simulink model "sampleModel1946"  (R2023a)
settings: Solver=VariableStepAuto  StartTime=0.0  StopTime=10.0  RelTol=1e-3
libraries: hdlsllib x1
settings Model: Creator=user1  LastModifiedBy=user1

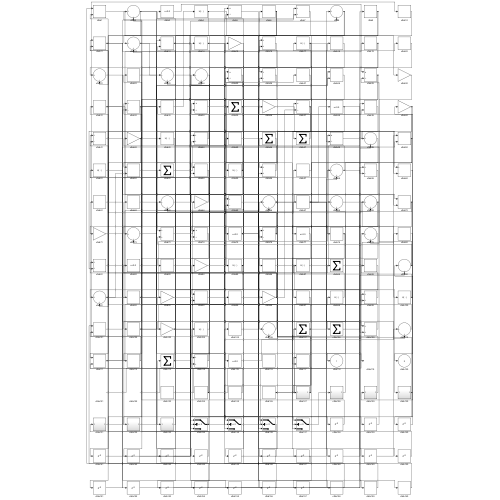
[thumbnail: Simulink's stored preview of the top-level diagram]
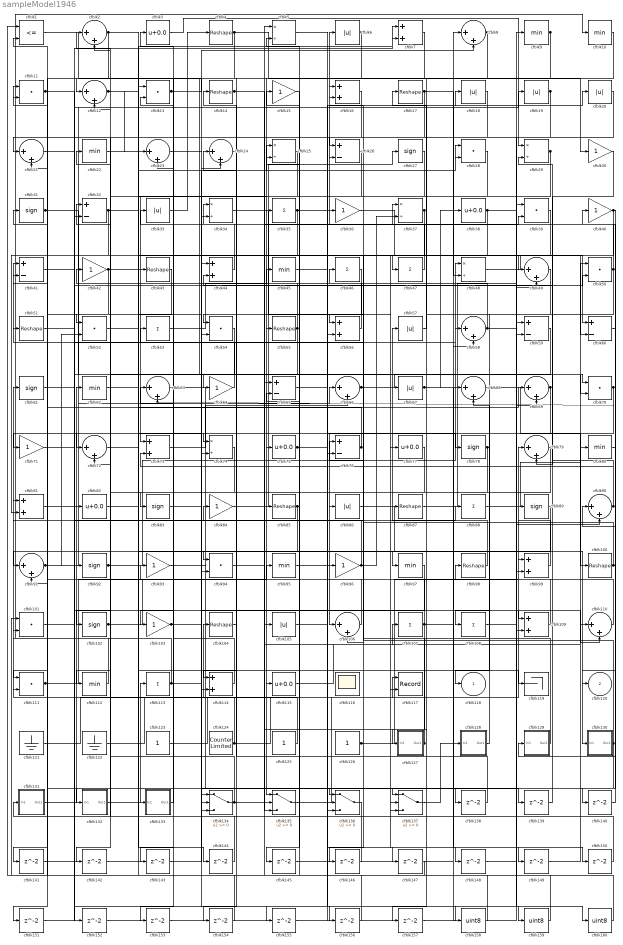
== system sampleModel1946 ==
  cfblk1 : RelationalOperator  Operator=<=  OutDataTypeStr=boolean  InputSameDT=off
  cfblk{9..10,22,45,62,80,95,97,112} (9 alike) : MinMax
  cfblk{4,14,17,43,51,55,85,87,98,100,104} (11 alike) : Reshape
  cfblk{11,13,28,39,50,52,54,70,94,101,111} (11 alike) : DotProduct  OutDataTypeStr=Inherit: Inherit via internal rule
  cfblk{27,31,61,78,83,89,92,102} (8 alike) : Signum
  cfblk{15,30,36,40,42,64,71,84,93,96,103} (11 alike) : Gain
  cfblk{6,18..20,33,57,67,86,105} (9 alike) : Abs  SaturateOnIntegerOverflow=off
  cfblk{2,8,12,21,23..24,49,58,63,66,68..69,72,79,90..91,106,110} (18 alike) : Sum  Inputs=|++
  cfblk{35,46..47,53,88,107..108,113} (8 alike) : Sum  Inputs=+
  cfblk{7,16,44,56,73,81,99,109,114} (9 alike) : Sum
  cfblk{3,38,75,77,82,115} (6 alike) : Bias  Bias=0.0  SaturateOnIntegerOverflow=off
  cfblk116 : Scope
      settings: Floating=on
  cfblk117 : Record  FileSettingsInternal="{\"entries\":[{\"content\":{\"excelSettings\":{\"content\":{},\"type\":\"Streamout.ExcelSettings\"}},\"type\":\"Streamout.FileSettingStorage\",\"uuid\":\"\"}],\"packageUris\":[\"http:\\/\\/schema.mathworks.com\\/mf0\\/streamout_blocks\\/R2020a\"],\"version\":\"1.0\"}"  Layout=[1 1]  SignalsInternal="{\"entries\":[{\"content\":{\"signals\":[{\"content\":{\"blockPath\":[],\"dimensions\":[1],\"domain\":\"\",\"lineColor\":\"#a2142f\",\"plots\":[1],\"port\":1,\"sid\":[\"\"],\"signalID\":5422,\"signalName\":\"cfblk135\"},\"type\":\"RecordBlkView.Signal\",\"uuid\":\"\"},{\"content\":{\"blockPath\":[],\"dimensions\":[1],\"domain\":\"\",\"lineColor\":\"#139fff\",\"plots\":[1],\"port\":2,\"sid\":[\"\"],\"signalID\":5426,\"signalName\":\"cfblk40\"},\"type\":\"RecordBlkView.Signal\",\"uuid\":\"\"}]},\"type\":\"RecordBlkView.InputSignals\",\"uuid\":\"\"}],\"packageUris\":[\"http:\\/\\/schema.mathworks.com\\/mf0\\/streamout_blocks\\/R2020a\"],\"version\":\"1.0\"}"  VisualizationBindings="{\"xyplotplugin\":{\"info\":[{\"series\":[{\"bindingParametersList\":[{\"parameter\":\"X-Axis\",\"signalID\":5422,\"signalName\":\"cfblk135\"},{\"parameter\":\"Y-Axis\",\"signalID\":5426,\"signalName\":\"cfblk40\"}],\"seriesID\":32701}],\"subplotID\":1}]}}"  CompatibilityTag=XY  st=-1
  cfblk119 : Terminator
  cfblk121 : Ground
  cfblk122 : Ground
  cfblk123 : Constant  SampleTime=-1
  cfblk124 : hdlsllib/Sources/Counter Limited  uplimit=7  tsamp=-1
  cfblk125 : Constant  SampleTime=-1
  cfblk126 : Constant  SampleTime=-1
  cfblk127 : Subsystem
      settings: LibrarySourceBlock=|
      | hdlsllib/Ports &
      | Subsystems/Subsystem
  cfblk128 : Subsystem
      settings: LibrarySourceBlock=|
      | hdlsllib/Ports &
      | Subsystems/Subsystem
  cfblk129 : Subsystem
      settings: LibrarySourceBlock=|
      | hdlsllib/Ports &
      | Subsystems/Subsystem
  cfblk130 : Subsystem
      settings: LibrarySourceBlock=|
      | hdlsllib/Ports &
      | Subsystems/Subsystem
  cfblk131 : Subsystem
      settings: LibrarySourceBlock=|
      | hdlsllib/Ports &
      | Subsystems/Subsystem
  cfblk132 : Subsystem
      settings: LibrarySourceBlock=|
      | hdlsllib/Ports &
      | Subsystems/Subsystem
  cfblk133 : Subsystem
      settings: LibrarySourceBlock=|
      | hdlsllib/Ports &
      | Subsystems/Subsystem
  cfblk{134..137} (4 alike) : Switch  SaturateOnIntegerOverflow=off  InputSameDT=off
  cfblk{138..157} (20 alike) : Delay  SampleTime=1
  cfblk158 : DataTypeConversion  OutDataTypeStr=uint8  SaturateOnIntegerOverflow=off  RndMeth=Floor
  cfblk159 : DataTypeConversion  OutDataTypeStr=uint8  SaturateOnIntegerOverflow=off  RndMeth=Floor
  cfblk160 : DataTypeConversion  OutDataTypeStr=uint8  SaturateOnIntegerOverflow=off  RndMeth=Floor
  cfblk{5,25,29,34,37,48,74} (7 alike) : Product  Inputs=*/  RndMeth=Zero  SaturateOnIntegerOverflow=on
  cfblk{26,32,41,59..60,65,76} (7 alike) : Sum  Inputs=+-
  cfblk118 : Outport  VectorParamsAs1DForOutWhenUnconnected=off
  cfblk120 : Outport  Port=2  VectorParamsAs1DForOutWhenUnconnected=off
  wires:
  cfblk126/1 -> cfblk98/1, cfblk58/2
  cfblk33/1 -> cfblk4/1
  cfblk86/1 -> cfblk130/1(In1)
  cfblk12/1 -> cfblk23/1, cfblk70/2
  cfblk81/1 -> cfblk66/1
  cfblk4/1 -> cfblk106/1, cfblk30/1
  cfblk69/1 -> cfblk86/1, cfblk137/3
  cfblk35/1 -> cfblk78/1, cfblk154/1
  cfblk7/1 -> cfblk135/1
  cfblk13/1 -> cfblk8/2, cfblk138/1
  cfblk136/1 -> cfblk131/1(In1)
  cfblk3/1 -> cfblk29/1
  cfblk90/1 -> cfblk44/2, cfblk73/2
  cfblk25/1 -> cfblk73/1
  cfblk49/1 -> cfblk108/1
  cfblk84/1 -> cfblk27/1
  cfblk91/1 -> cfblk19/1, cfblk52/2
  cfblk40/1 -> cfblk129/1(In1), cfblk117/2
  cfblk112/1 -> cfblk10/1
  cfblk47/1 -> cfblk34/1
  cfblk79/1 -> cfblk106/2
  cfblk125/1 -> cfblk61/1
  cfblk44/1 -> cfblk33/1
  cfblk46/1 -> cfblk85/1
  cfblk131/1(Out1) -> cfblk62/1
  cfblk50/1 -> cfblk6/1, cfblk127/1(In1), cfblk157/1
  cfblk135/1 -> cfblk117/1
  cfblk63/1 -> cfblk115/1
  cfblk8/1 -> cfblk47/1, cfblk76/2
  cfblk16/1 -> cfblk91/1
  cfblk64/1 -> cfblk41/1
  cfblk43/1 -> cfblk132/1(In1)
  cfblk57/1 -> cfblk17/1
  cfblk115/1 -> cfblk80/1
  cfblk133/1(Out1) -> cfblk63/1
  cfblk92/1 -> cfblk48/1, cfblk67/1
  cfblk93/1 -> cfblk137/1
  cfblk122/1 -> cfblk104/1
  cfblk48/1 -> cfblk60/1
  cfblk100/1 -> cfblk46/1, cfblk40/1
  cfblk17/1 -> cfblk48/2, cfblk97/1, cfblk135/3
  cfblk37/1 -> cfblk71/1, cfblk146/1
  cfblk38/1 -> cfblk83/1, cfblk150/1
  cfblk9/1 -> cfblk12/1, cfblk74/1
  cfblk58/1 -> cfblk16/1, cfblk160/1
  cfblk123/1 -> cfblk79/1
  cfblk6/1 -> cfblk23/2, cfblk103/1, cfblk21/2
  cfblk70/1 -> cfblk63/2, cfblk141/1
  cfblk132/1(Out1) -> cfblk113/1
  cfblk129/1(Out1) -> cfblk51/1
  cfblk95/1 -> cfblk36/1
  cfblk78/1 -> cfblk118/1, cfblk137/2
  cfblk82/1 -> cfblk133/1(In1)
  cfblk137/1 -> cfblk128/1(In1)
  cfblk29/1 -> cfblk55/1, cfblk136/3
  cfblk98/1 -> cfblk57/1
  cfblk18/1 -> cfblk114/1
  cfblk31/1 -> cfblk96/1, cfblk64/1
  cfblk24/1 -> cfblk94/1
  cfblk88/1 -> cfblk50/1
  cfblk87/1 -> cfblk9/1
  cfblk111/1 -> cfblk95/1, cfblk50/2
  cfblk61/1 -> cfblk58/1
  cfblk94/1 -> cfblk39/2
  cfblk28/1 -> cfblk75/1
  cfblk1/1 -> cfblk24/2
  cfblk20/1 -> cfblk26/1
  cfblk104/1 -> cfblk84/1
  cfblk54/1 -> cfblk102/1
  cfblk110/1 -> cfblk42/1
  cfblk73/1 -> cfblk66/2
  cfblk124/1 -> cfblk59/1, cfblk53/1, cfblk101/2
  cfblk68/1 -> cfblk100/1
  cfblk67/1 -> cfblk109/1, cfblk20/1, cfblk38/1, cfblk149/1
  cfblk107/1 -> cfblk135/2, cfblk99/1, cfblk81/1
  cfblk77/1 -> cfblk134/2
  cfblk99/1 -> cfblk89/1
  cfblk39/1 -> cfblk56/1
  cfblk114/1 -> cfblk13/2
  cfblk62/1 -> cfblk119/1
  cfblk55/1 -> cfblk114/2, cfblk2/2, cfblk54/1
  cfblk96/1 -> cfblk11/1, cfblk37/2, cfblk41/2, cfblk22/1
  cfblk103/1 -> cfblk69/1, cfblk28/2
  cfblk109/1 -> cfblk15/1
  cfblk130/1(Out1) -> cfblk93/1, cfblk151/1
  cfblk26/1 -> cfblk72/1
  cfblk19/1 -> cfblk59/2, cfblk142/1
  cfblk27/1 -> cfblk52/1
  cfblk22/1 -> cfblk43/1
  cfblk97/1 -> cfblk134/3
  cfblk23/1 -> cfblk136/1
  cfblk128/1(Out1) -> cfblk68/2
  cfblk121/1 -> cfblk105/1
  cfblk71/1 -> cfblk109/2
  cfblk74/1 -> cfblk112/1
  cfblk42/1 -> cfblk111/1, cfblk12/2, cfblk74/2
  cfblk66/1 -> cfblk70/1, cfblk148/1
  cfblk14/1 -> cfblk110/2, cfblk139/1
  cfblk32/1 -> cfblk7/1, cfblk49/1, cfblk81/2, cfblk54/2
  cfblk45/1 -> cfblk18/1
  cfblk127/1(Out1) -> cfblk76/1, cfblk82/1
  cfblk83/1 -> cfblk25/1
  cfblk34/1 -> cfblk77/1
  cfblk101/1 -> cfblk87/1
  cfblk134/1 -> cfblk32/1, cfblk107/1
  cfblk60/1 -> cfblk120/1
  cfblk108/1 -> cfblk90/2
  cfblk11/1 -> cfblk16/2, cfblk155/1
  cfblk10/1 -> cfblk136/2
  cfblk72/1 -> cfblk28/1
  cfblk41/1 -> cfblk7/2
  cfblk113/1 -> cfblk11/2, cfblk156/1
  cfblk30/1 -> cfblk79/2
  cfblk106/1 -> cfblk14/1
  cfblk56/1 -> cfblk3/1
  cfblk102/1 -> cfblk65/1, cfblk26/2
  cfblk36/1 -> cfblk60/2
  cfblk53/1 -> cfblk45/1
  cfblk76/1 -> cfblk2/1, cfblk31/1
  cfblk51/1 -> cfblk92/1
  cfblk105/1 -> cfblk88/1
  cfblk2/1 -> cfblk21/1, cfblk99/2, cfblk35/1
  cfblk75/1 -> cfblk37/1, cfblk25/2, cfblk147/1
  cfblk85/1 -> cfblk65/2, cfblk91/2
  cfblk138/1 -> cfblk24/1
  cfblk139/1 -> cfblk29/2
  cfblk80/1 -> cfblk140/1
  cfblk140/1 -> cfblk90/1
  cfblk141/1 -> cfblk94/2
  cfblk142/1 -> cfblk34/2
  cfblk59/1 -> cfblk143/1
  cfblk143/1 -> cfblk44/1
  cfblk52/1 -> cfblk144/1
  cfblk144/1 -> cfblk134/1
  cfblk15/1 -> cfblk145/1
  cfblk145/1 -> cfblk68/1
  cfblk146/1 -> cfblk72/2
  cfblk147/1 -> cfblk1/1
  cfblk148/1 -> cfblk69/2
  cfblk149/1 -> cfblk110/1
  cfblk150/1 -> cfblk111/2
  cfblk151/1 -> cfblk32/2
  cfblk21/1 -> cfblk152/1
  cfblk152/1 -> cfblk39/1
  cfblk89/1 -> cfblk153/1
  cfblk153/1 -> cfblk8/1
  cfblk154/1 -> cfblk13/1
  cfblk155/1 -> cfblk56/2
  cfblk156/1 -> cfblk1/2
  cfblk157/1 -> cfblk49/2
  cfblk5/1 -> cfblk158/1
  cfblk158/1 -> cfblk101/1
  cfblk65/1 -> cfblk159/1
  cfblk159/1 -> cfblk5/1
  cfblk160/1 -> cfblk5/2

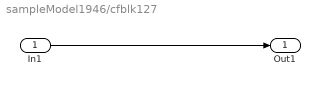
== system sampleModel1946/cfblk127 ==
  In1 : Inport
  Out1 : Outport
  wires:
  In1/1 -> Out1/1

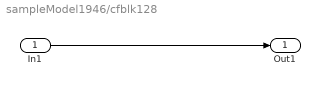
== system sampleModel1946/cfblk128 ==
  In1 : Inport
  Out1 : Outport
  wires:
  In1/1 -> Out1/1

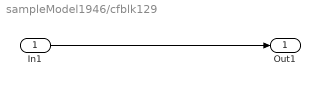
== system sampleModel1946/cfblk129 ==
  In1 : Inport
  Out1 : Outport
  wires:
  In1/1 -> Out1/1

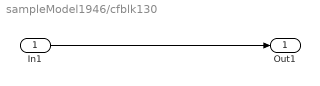
== system sampleModel1946/cfblk130 ==
  In1 : Inport
  Out1 : Outport
  wires:
  In1/1 -> Out1/1

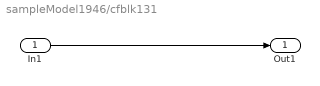
== system sampleModel1946/cfblk131 ==
  In1 : Inport
  Out1 : Outport
  wires:
  In1/1 -> Out1/1

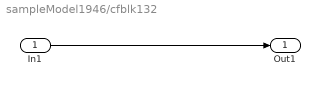
== system sampleModel1946/cfblk132 ==
  In1 : Inport
  Out1 : Outport
  wires:
  In1/1 -> Out1/1

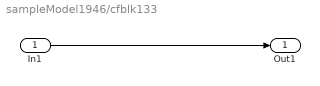
== system sampleModel1946/cfblk133 ==
  In1 : Inport
  Out1 : Outport
  wires:
  In1/1 -> Out1/1
